simulink model "ejemplo_ecuacion"  (R2023a)
settings: Solver=VariableStepAuto  StartTime=0.0  StopTime=10.0  RelTol=1e-3
settings Model: Creator=Nacho Andrade  LastModifiedBy=Nacho Andrade

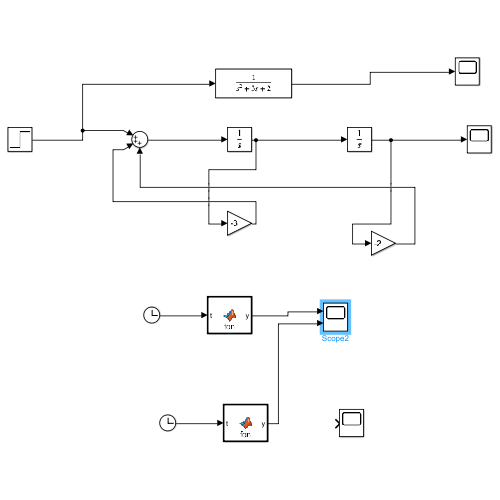
[thumbnail: Simulink's stored preview of the top-level diagram]
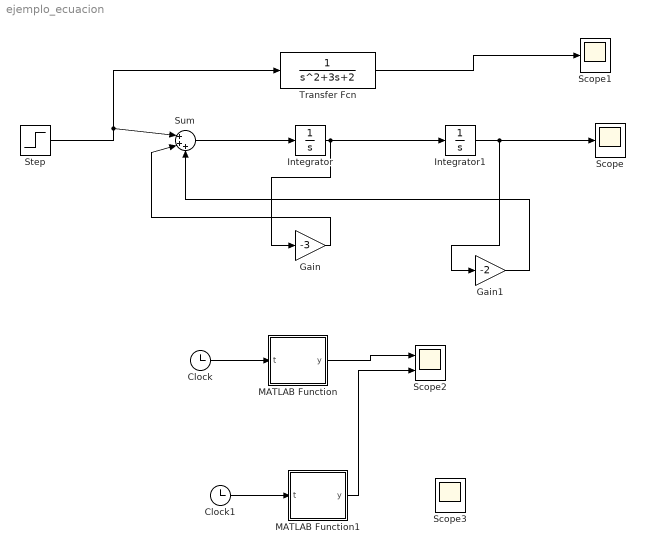
== system ejemplo_ecuacion ==
  Clock : Clock
  Clock1 : Clock
  Gain : Gain  Gain=-3
  Gain1 : Gain  Gain=-2
  Integrator : Integrator
  Integrator1 : Integrator
  MATLAB Function : MATLAB Function  TreatAsAtomicUnit=on
  MATLAB Function1 : MATLAB Function  TreatAsAtomicUnit=on
  Scope : Scope
  Scope1 : Scope
  Scope2 : Scope  NumInputPorts=2
  Scope3 : Scope
  Step : Step  Before=1  After=3  SampleTime=0
  Sum : Sum  Inputs=|+++
  Transfer Fcn : TransferFcn  Denominator=[1 3 2]
  wires:
  Integrator/1 -> Gain/1, Integrator1/1
  Sum/1 -> Integrator/1
  Step/1 -> Transfer Fcn/1, Sum/1
  Integrator1/1 -> Scope/1, Gain1/1
  Gain/1 -> Sum/2
  Gain1/1 -> Sum/3
  Transfer Fcn/1 -> Scope1/1
  Clock/1 -> MATLAB Function/1(t)
  MATLAB Function/1(y) -> Scope2/1
  Clock1/1 -> MATLAB Function1/1(t)
  MATLAB Function1/1(y) -> Scope2/2

== matlab function ejemplo_ecuacion/MATLAB Function ==
  data: t input; y output
function y = fcn(t)

y = (-216*exp(1)/289)*exp(-t) + (216*exp(1)/17).*t.*exp(-t) + (216*exp(1)/289)*exp(-18*t);

== matlab function ejemplo_ecuacion/MATLAB Function1 ==
  data: t input; y output
function y = fcn(t)

y = 12*t.*exp(1-t);
